simulink model "bmw_new"  (R2020a)
settings: Solver=VariableStepAuto  StartTime=0.0  StopTime=10.0  RelTol=1e-3
settings Model: Creator=UBY 00  LastModifiedBy=muham

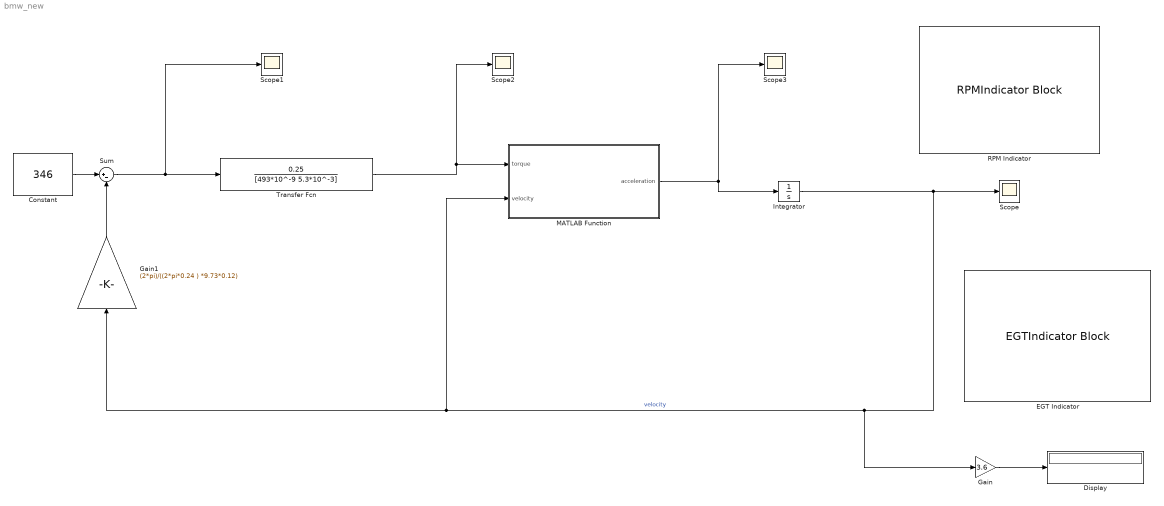
== system bmw_new ==
  Constant : Constant  Value=346
  Display : Display
  EGT Indicator : EGTIndicatorBlock
  Gain : Gain  Gain=3.6
  Gain1 : Gain  Gain=(2*pi)/((2*pi*0.24 ) *9.73*0.12)
  Integrator : Integrator
  MATLAB Function : MATLAB Function  TreatAsAtomicUnit=on
  RPM Indicator : RPMIndicatorBlock
  Scope{,1..3} (4 alike) : Scope
  Sum : Sum  Inputs=|+-
  Transfer Fcn : TransferFcn  Numerator=[0.25]  Denominator=[493*10^-9 5.3*10^-3]
  wires:
  MATLAB Function/1(acceleration) -> Integrator/1, Scope3/1
  Integrator/1 -> Gain/1, MATLAB Function/2(velocity), Gain1/1, Scope/1  "velocity"
  Constant/1 -> Sum/1
  Sum/1 -> Scope1/1, Transfer Fcn/1
  Gain/1 -> Display/1
  Transfer Fcn/1 -> Scope2/1, MATLAB Function/1(torque)
  Gain1/1 -> Sum/2

== matlab function bmw_new/MATLAB Function ==
  data: torque input; acceleration output; velocity input
function acceleration = bmw_i8(torque,velocity)

acceleration=(40.5*torque*0.7-413-0.3381*velocity.^2)/(2108)
end
